simulink model "Expt_2_2"  (R2018b)
settings: Solver=VariableStepAuto  StartTime=0.0  StopTime=100000  RelTol=1e-3
settings Model: Creator=HP  LastModifiedBy=HP
settings DebuggingCC: LibraryContextMissingDiagnostic=none
settings SFSimCC: SimUseLocalCustomCode=off
settings RTWCC: RTWUseLocalCustomCode=off

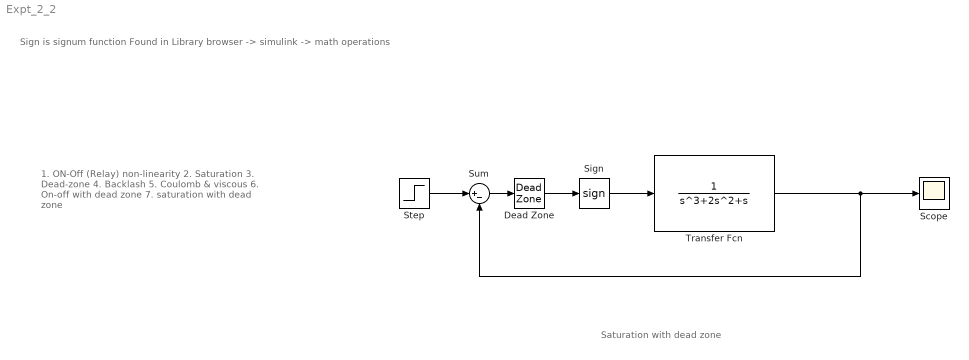
== system Expt_2_2 ==
  note: Saturation with dead zone
  note: 1. ON-Off (Relay) non-linearity
      | 2. Saturation
      | 3. Dead-zone
      | 4. Backlash
      | 5. Coulomb & viscous
      | 6. On-off with dead zone
      | 7. saturation with dead zone
  note: Sign is signum function
      | Found in Library browser -> simulink -> math operations
  Dead Zone : DeadZone  SaturateOnIntegerOverflow=on
  Scope : Scope
  Sign : Signum
  Step : Step  SampleTime=0
  Sum : Sum  Inputs=|+-
  Transfer Fcn : TransferFcn  Denominator=[1 2 1 0]
  wires:
  Transfer Fcn/1 -> Sum/2, Scope/1
  Step/1 -> Sum/1
  Sign/1 -> Transfer Fcn/1
  Sum/1 -> Dead Zone/1
  Dead Zone/1 -> Sign/1
